simulink model "ssc_car_fuel_cell_1motor"  (R2026a)
settings: Solver=daessc  StopTime=195  FixedStep=1e-3  AbsTol=1e-3
InitFcn:
  | %Vehicle = sm_car_vehcfg_checkConfig(Vehicle);
undefined symbols (not defined in the file): Control, Driver, Init, Maneuver1, Vehicle
libraries: fl_lib x93, nesl_utility x38, GasN_lib x21, sdl_lib x10, simulink_extras x6, SimscapeFluids_lib x6, simulink x5, customMath_lib x5, slpidlib x4, ee_lib x3, autolibshared x2, sl_discontinuities x2
(part 2 of 4)

== system ssc_car_fuel_cell_1motor/Fuel Cell 1 Motor/Regen Torque Limit/Mech to Elec Power Estimate ==
  note: Check if Motoring
      | or Generating
  note: Using an Efficiency Map, we can estimate the
      | Electric Power from the Mechanical  Torque Request.
  note: Pelec_req = Pmech_req*Eff^k,
      | k = -1 if Motoring >= 0,
      | k = 1 if Generating < 0
  MotTrqCmd : Inport
  MotSpd : Inport  Port=2
  Abs : Abs  ZeroCross=off  SaturateOnIntegerOverflow=off
  Abs1 : Abs  ZeroCross=off  SaturateOnIntegerOverflow=off
  Constant1 : Constant  Value=-1  SampleTime=0
  Constant2 : Constant  SampleTime=0
  Eff Map : Lookup_n-D  BreakpointsForDimension1=Control.MotorA1.LossTable.w.Value  BreakpointsForDimension2=Control.MotorA1.LossTable.trq.Value  Table=Control.MotorA1.LossTable.efficiency.Value  ExtrapMethod=Clip  UseLastTableValue=on  InternalRulePriority=Speed  OutDataTypeStr=Inherit: Inherit from 'Table data'  RndMeth=Simplest
      settings: InputPortMap=u0,u1
  Gain1 : Gain  Gain=1/100
  Math Function : Math  Operator=pow  SignedPower=on  OutputSignalType=real
  Product : Product
  Product3 : Product
  Product4 : Product
  Scope : Scope  NumInputPorts=4
      settings: ActiveDisplayYMinimum=84.125  ActiveDisplayYMaximum=92.875  DataLoggingVariableName=ScopeData2
  Switch2 : Switch  ZeroCross=off  SaturateOnIntegerOverflow=off  InputSameDT=off
  rads_to_rpm : Gain  Gain=30/pi
  MotPwrElecReq : Outport  VectorParamsAs1DForOutWhenUnconnected=off
  Eff2k : Outport  Port=2  VectorParamsAs1DForOutWhenUnconnected=off
  wires:
  Product3/1 -> Product4/1
  Switch2/1 -> Math Function/2
  Constant1/1 -> Switch2/1
  Constant2/1 -> Switch2/3
  Eff Map/1 -> Gain1/1, Scope/1
  Abs/1 -> Eff Map/1
  Gain1/1 -> Math Function/1
  Math Function/1 -> Eff2k/1, Product4/2
  Product4/1 -> MotPwrElecReq/1, Scope/2
  Abs1/1 -> Eff Map/2
  rads_to_rpm/1 -> Abs/1
  Product/1 -> Switch2/2
  MotSpd/1 -> Product3/1, Product/1, Scope/3, rads_to_rpm/1
  MotTrqCmd/1 -> Product3/2, Product/2, Scope/4, Abs1/1

== system ssc_car_fuel_cell_1motor/Fuel Cell 1 Motor/Regen Torque Limit/Torque Limit ==
  MotTrq : Inport
  MotSpd : Inport  Port=2
  Gain : Gain  Gain=-1
  MaxMotTrqVsSpd : Lookup_n-D  NumberOfTableDimensions=1  BreakpointsForDimension1=Control.MotorA1.TorqueSpd.w.Value  Table=Control.MotorA1.TorqueSpd.trq.Value  ExtrapMethod=Clip  UseLastTableValue=on  InternalRulePriority=Speed  OutDataTypeStr=Inherit: Inherit from 'Table data'  RndMeth=Simplest
  Saturation Dynamic : sl_discontinuities/Saturation Dynamic  OutMin=[]  OutMax=[]  OutDataTypeStr=Inherit: Same as second input  OutDataType=fixdt(1, 16)  OutScaling=2^-10  DoSatur=off
  rads_to_rpm : Gain  Gain=30/pi
  MotReqCmd : Outport  VectorParamsAs1DForOutWhenUnconnected=off
  wires:
  MotTrq/1 -> Saturation Dynamic/2
  MotSpd/1 -> rads_to_rpm/1
  MaxMotTrqVsSpd/1 -> Gain/1, Saturation Dynamic/1
  rads_to_rpm/1 -> MaxMotTrqVsSpd/1
  Gain/1 -> Saturation Dynamic/3
  Saturation Dynamic/1 -> MotReqCmd/1

== system ssc_car_fuel_cell_1motor/Fuel Cell 1 Motor/Susp/Steer ==
  Bus Creator : BusCreator  Inputs=1
  Constant : Constant  Value=0
  Steer : Outport  VectorParamsAs1DForOutWhenUnconnected=off
  wires:
  Bus Creator/1 -> Steer/1  "Steer"
  Constant/1 -> Bus Creator/1  "iMotor"

== system ssc_car_fuel_cell_1motor/Vehicle/Powertrain/Driveline ==
  Differential : sdl_lib/Gears/Differential  driveshaft_location=2  cd_ratio=Vehicle.Powertrain.Driveline.DifferentialA1.ratio.Value  friction_model=1  efficiency=[.85, .92]  temperature_TLU=[280, 300, 320] K  efficiency_ss_TLU=[.95, .9, .85]  efficiency_cd_TLU=[.95, .9, .85]  pwr_thr=[.001, .001] W  mu_visc=[0, 0] N*m/(rad/s)  model_inertia=0  sun_inertia=1e-10 kg*m^2  sun_radius=0.01 m  carrier_inertia=0.001 kg*m^2  planet_inertia=0.001 kg*m^2  planet_mass=1e-10 kg  thermal_mass=50 J/K  T_init=300 K
  Gear Box : fl_lib/Mechanical/Mechanisms/Gear Box  ratio=Vehicle.Powertrain.Driveline.GearboxA1.ratio.Value  t_in_specify=off  t_in_priority=None  t_in=0 N*m  t_in_nominal_specify=off  t_in_nominal_value=1  t_in_nominal_unit=N*m  t_out_specify=off  t_out_priority=None  t_out=0 N*m  t_out_nominal_specify=off  t_out_nominal_value=1  t_out_nominal_unit=N*m
  Sensor Speed and Power : Subsystem
      mask Display: disp('S')
  Simscape Bus : SimscapeBus  HierarchyStrings=ShaftA1
  L1 : PMIOPort  Side=Left
  Sh : PMIOPort  Port=2  Side=Left
  R1 : PMIOPort  Port=3  Side=Right
  FR1 : PMIOPort  Port=4  Side=Right
  connections:
  Gear Box/LConn1 -- Sensor Speed and Power/RConn1
  Simscape Bus/LConn1 -- Sensor Speed and Power/LConn1
  Differential/RConn2 -- L1/RConn1
  Sh/RConn1 -- Simscape Bus/RConn1
  Differential/RConn1 -- FR1/RConn1 -- R1/RConn1
  Differential/LConn1 -- Gear Box/RConn1

== system ssc_car_fuel_cell_1motor/Vehicle/Powertrain/FuelCell1Motor ==
  In Bus Element : Inport  PortName=CtrlBus  Element=FuelCell
  In Bus Element4 : Inport  PortName=CtrlBus  Element=MotorA1.trqCmd
  In Bus Element1 : Inport  Port=2  PortName=VehBus  Element=Body.CG
  Ambient Temperature : fl_lib/Thermal/Thermal Sources/Temperature Source  temperature=300 K
  Battery : Subsystem  VariantControl=0  mask{Battery=Power.Battery}
      mask prompts: Battery "Battery (structure)"
      mask Display: image('sm_car_vehicle_power_battery_system_IMAGE.png');
  Electrical Reference1 : fl_lib/Electrical/Electrical Elements/Electrical Reference
  Fuel Cell : Subsystem  VariantControl=0  mask{FuelCell=Power.FuelCell}
      mask prompts: FuelCell "Fuel Cell (structure)"
      mask Display: image('sm_car_vehicle_power_fuel_cell_converter_IMAGE.png');
  Motor A1 : Subsystem  mask{Motor=Power.MotorA1}
      mask prompts: Motor "Motor (structure)"
      mask Display: image('sm_car_vehicle_power_emotor_simplified_IMAGE.png');
  Simscape Bus : SimscapeBus  HierarchyStrings=ShaftA1
  Thermal System : Subsystem  mask{Cooling=Power.Cooling}
      mask prompts: Cooling "Cooling (structure)"
      mask Display: image('sm_car_vehicle_power_cooling_active1loop_IMAGE.png');
  Shafts : PMIOPort  Side=Left
  Out Bus Element : Outport  PortName=OutP  Element=FuelCell
  Out Bus Element1 : Outport  PortName=OutP  Element=MotorA1
  Out Bus Element2 : Outport  PortName=OutP  Element=Battery
  Out Bus Element3 : Outport  PortName=OutP  Element=Thermal
  wires:
  Battery/1(m) -> Out Bus Element2/1
  Thermal System/1(m) -> Out Bus Element3/1
  Fuel Cell/1(m) -> Out Bus Element/1
  Motor A1/1(m) -> Out Bus Element1/1
  In Bus Element1/1 -> Fuel Cell/2(VehBus)
  In Bus Element4/1 -> Motor A1/1(Tr)
  In Bus Element/1 -> Fuel Cell/1(CtrlBus)
  Fuel Cell/2(PBatt) -> Battery/1(PLoss)
  connections:
  Motor A1/LConn1 -- Fuel Cell/RConn1 -- Battery/RConn1
  Thermal System/LConn3 -- Battery/RConn4 -- Ambient Temperature/LConn1
  Thermal System/LConn2 -- Fuel Cell/RConn3 -- Battery/RConn3
  Motor A1/LConn3 -- Thermal System/LConn1
  Simscape Bus/RConn1 -- Shafts/RConn1
  Fuel Cell/RConn2 -- Electrical Reference1/LConn1 -- Motor A1/LConn2 -- Battery/RConn2
  Simscape Bus/LConn1 -- Motor A1/RConn1

== system ssc_car_fuel_cell_1motor/Vehicle/Powertrain/Driveline/Sensor Speed and Power ==
  Ideal Rotational Motion Sensor : fl_lib/Mechanical/Mechanical Sensors/Ideal Rotational Motion Sensor  reference=foundation.enum.MeasurementReference.difference  acceleration_port=false  velocity_port=true  position_port=true  wrap_angle=simscape.enum.onoff.off  offset=0 rad
  Ideal Torque Sensor : fl_lib/Mechanical/Mechanical Sensors/Ideal Torque Sensor
  Mechanical Rotational Reference : fl_lib/Mechanical/Rotational Elements/Mechanical Rotational Reference
  PS-Simulink Converter : nesl_utility/PS-Simulink Converter  PhysicalDomain=network_engine_domain  SubClassName=ps_output  LeftPortType=input  RightPortType=output  PseudoPeriodic=off  Frequencies=[]  VectorFormat=1-D array  Unit=N*m  AffineConversion=off
  PS-Simulink Converter1 : nesl_utility/PS-Simulink Converter  PhysicalDomain=network_engine_domain  SubClassName=ps_output  LeftPortType=input  RightPortType=output  PseudoPeriodic=off  Frequencies=[]  VectorFormat=1-D array  Unit=rad/s  AffineConversion=off
  Product : Product  RndMeth=Zero
  Terminator : Terminator
  W2kW : Gain  Gain=0.001
  B : PMIOPort  Side=Left
  F : PMIOPort  Port=2  Side=Right
  wires:
  W2kW/1 -> [Pm_vehicle]
  Product/1 -> W2kW/1
  PS-Simulink Converter/1 -> Product/1
  PS-Simulink Converter1/1 -> Product/2
  [Pm_vehicle] -> Terminator/1
  connections:
  Mechanical Rotational Reference/LConn1 -- Ideal Rotational Motion Sensor/RConn1
  Ideal Rotational Motion Sensor/LConn1 -- F/RConn1 -- Ideal Torque Sensor/RConn1
  B/RConn1 -- Ideal Torque Sensor/LConn1
  PS-Simulink Converter/LConn1 -- Ideal Torque Sensor/RConn2
  PS-Simulink Converter1/LConn1 -- Ideal Rotational Motion Sensor/RConn2

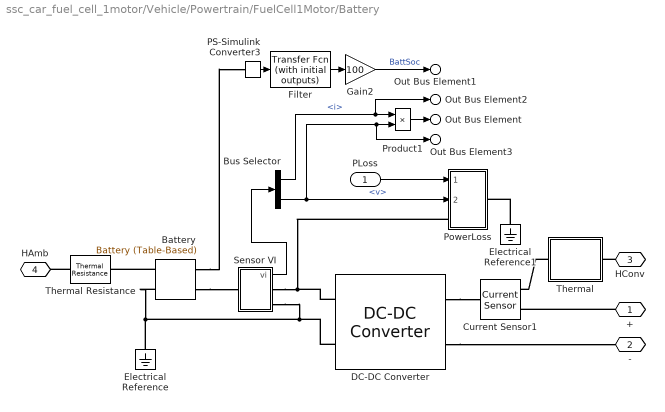
== system ssc_car_fuel_cell_1motor/Vehicle/Powertrain/FuelCell1Motor/Battery ==
  PLoss : Inport
  Battery : batteryecm_lib/Battery (Table-Based)  SOC_vec=Battery.vNoLoad.SOC.Value  T_dependence=simscape.enum.tablebattery.temperature_dependence.yes  prm_dir=simscape.enum.tablebattery.prm_dir.noCurrentDirectionality  T_vec=Battery.vNoLoad.T.Value K  V0_mat=Battery.vNoLoad.V0.Value V  V0_vec=[3.1, 3.27, 3.31, 3.5] V  V_range=[0, inf] V  R0_mat=Battery.rTerminal.R0.Value Ohm  R0_vec=[.015, .017, .012, .013] Ohm  R0_dis_mat=[.03, .015, .002; .04, .017, .008; .039, .012, .006; .027, .013, .021] Ohm  R0_dis_vec=[.015, .017, .012, .013] Ohm  R0_ch_mat=[.03, .015, .002; .04, .017, .008; .039, .012, .006; .027, .013, .021] Ohm  R0_ch_vec=[.015, .017, .012, .013] Ohm  AH=Battery.AhTable.Ah.Value hr*A  prm_leak=1  Rleak_vec=ones(size(Battery.vNoLoad.T.Value))*10000 Ohm  Rleak=7e3 Ohm  extrapolation_option=simscape.enum.extrapolation.linear  SOC_port=simscape.enum.tablebattery.enable.yes  prm_dyn=1  R1_mat=[.089, .076, .01; .042, .022, .099; .019, .007, .002; .051, .043, .029] Ohm  R1_vec=[.076, .022, .007, .043] Ohm  tau1_mat=[44, 148, 235; 93, 110, 1000; 19, 27, 133; .5, 22, 3] s  tau1_vec=[148, 110, 27, 22] s  R2_mat=[.014, .382, .407; .028, .006, .007; .014, .007, .006; .333, .956, .912] Ohm  R2_vec=[.382, .006, .007, .956] Ohm  tau2_mat=[1, 44, 5644; 11, 24, 506; 2, 14, 330; 3310, 13419, 30216] s  tau2_vec=[44, 24, 14, 13419] s  R3_mat=[.014, .382, .407; .028, .006, .007; .014, .007, .006; .333, .956, .912] Ohm  R3_vec=[.382, .006, .007, .956] Ohm  tau3_mat=[1, 44, 5644; 11, 24, 506; 2, 14, 330; 3310, 13419, 30216] s  tau3_vec=[44, 24, 14, 13419] s  R4_mat=[.014, .382, .407; .028, .006, .007; .014, .007, .006; .333, .956, .912] Ohm  R4_vec=[.382, .006, .007, .956] Ohm  tau4_mat=[1, 44, 5644; 11, 24, 506; 2, 14, 330; 3310, 13419, 30216] s  tau4_vec=[44, 24, 14, 13419] s  R5_mat=[.014, .382, .407; .028, .006, .007; .014, .007, .006; .333, .956, .912] Ohm  R5_vec=[.382, .006, .007, .956] Ohm  tau5_mat=[1, 44, 5644; 11, 24, 506; 2, 14, 330; 3310, 13419, 30216] s  tau5_vec=[44, 24, 14, 13419] s  prm_fade=simscape.enum.tablebattery.prm_fade.equations  N0=100  dV0=0  dR0=0  dAH=0  dRleak=0  dR1=0  dR2=0  dR3=0  dR4=0  dR5=0  N0vec=[100, 200, 300]  Tfadevec=[298.15, 323.15] K  dV0vec=[0, 0, 0]  dR0vec=[0, 0, 0]  dAHvec=[0, 0, 0]  dRleakvec=[0, 0, 0]  dR1vec=[0, 0, 0]  dR2vec=[0, 0, 0]  dR3vec=[0, 0, 0]  dR4vec=[0, 0, 0]  dR5vec=[0, 0, 0]  dV0mat=[0, 0; 0, 0; 0, 0]  dR0mat=[0, 0; 0, 0; 0, 0]  dAHmat=[0, 0; 0, 0; 0, 0]  dRleakmat=[0, 0; 0, 0; 0, 0]  dR1mat=[0, 0; 0, 0; 0, 0]  dR2mat=[0, 0; 0, 0; 0, 0]  dR3mat=[0, 0; 0, 0; 0, 0]  dR4mat=[0, 0; 0, 0; 0, 0]  dR5mat=[0, 0; 0, 0; 0, 0]  prm_age_modeling=simscape.enum.tablebattery.prm_age_modeling.equation  storage_dt_age_vec=[0] d  storage_T_age_vec=[273] K  prm_age_OCV=simscape.enum.tablebattery.prm_age_OCV.OCV  OCV_age=0.9  SOC_age=0.6  prm_age_resistance=simscape.enum.tablebattery.prm_age.disabled  OCV_scaling_age_resistance=2.2134e6  OCV_offset_age_resistance=1.632e6  temp_exp_age_resistance=0.515833569 V  t_exp_age_resistance=0.75  T_age_vec_resistance=[273.15, 298.15, 323.15] K  dt_age_vec_resistance=[90, 180, 270, 360] d  dR0_age_vec=[0, 0, 0]  t_meas_dR0_age=100 d  dR0_age_mat=[0, 0, 0; 0, 0, 0; 0, 0, 0; 0, 0, 0]  prm_age_capacity=simscape.enum.tablebattery.prm_age.disabled  OCV_scaling_age_capacity=1.5097e07  OCV_offset_age_capacity=8.3625e06  temp_exp_age_capacity=0.6011 V  t_exp_age_capacity=0.75  T_age_vec_capacity=[273.15, 298.15, 323.15] K  dt_age_vec_capacity=[90, 180, 270, 360] d  dAH_age_vec=[0, 0, 0]  t_meas_dAH_age=100 d  dAH_age_mat=[0, 0, 0; 0, 0, 0; 0, 0, 0; 0, 0, 0]  thermal_port=simscape.enum.thermaleffects.model  temperature=Battery.TInit.Value K  thermal_mass=Battery.mThermal.Value J/K  i_specify=on  i_priority=None  i=1e-3 A  i_nominal_specify=off  i_nominal_value=1  i_nominal_unit=A  v_specify=off  v_priority=None  v=0 V  v_nominal_specify=off  v_nominal_value=1  v_nominal_unit=V  stateOfCharge_specify=on  stateOfCharge_priority=High  stateOfCharge=Battery.SOCInit.Value  stateOfCharge_nominal_specify=off  stateOfCharge_nominal_value=1  stateOfCharge_nominal_unit=1  num_cycles_specify=off  num_cycles_priority=High  num_cycles=0  num_cycles_nominal_specify=off  num_cycles_nominal_value=1  num_cycles_nominal_unit=1  cell_temperature_specify=on  cell_temperature_priority=High  cell_temperature=Battery.TInit.Value K  cell_temperature_nominal_specify=off  cell_temperature_nominal_value=1  cell_temperature_nominal_unit=K
  Bus Selector : BusSelector  OutputSignals=i,v
  Current Sensor1 : fl_lib/Electrical/Electrical Sensors/Current Sensor
  DC-DC Converter : ee_lib/Semiconductors & Converters/Converters/DC-DC Converter  Vref_option=ee.enum.converters.voltageref.internal  v_ref="Battery.Converter.vRef.Value  V"  P_rated=Battery.Converter.power.Value W  droop_enabled=true  droop_param=1  droop=Battery.Converter.droopVpA.Value V/A  droop_percent=2  Vref_droop=10 V  reversible=1  G_diode=1e-6 1/Ohm  P_fixed=Battery.Converter.lossFixed.Value W  losses_option=ee.enum.converters.lossesOption.proportionalToSquaredCurrent  eff_rated=80  tableOption=ee.enum.converters.lossTableOption.current  i_eff_vec=[1, 2, 3, 4] A  v_eff_vec=[15, 30, 45] V  eff_vec=[90, 80, 70, 60]  eff_2D_table=[90, 85, 80; 80, 75, 70; 70, 65, 60; 60, 55, 50]  model_dynamics=0  tau=0.02 s  v_ini=650 V  v1_min=1 V  R1=1000 Ohm  R2=1000 Ohm  T_eff_vec=[280, 300, 320] K  eff_3D_table=repmat([66; 76; 80; 74], 1, 3, 3)  thermal_mass=100 J/K  initial_temperature=298.15 K
  Electrical Reference : fl_lib/Electrical/Electrical Elements/Electrical Reference
  Electrical Reference1 : fl_lib/Electrical/Electrical Elements/Electrical Reference
  Filter : simulink_extras/Additional Linear/Transfer Fcn (with initial outputs)  N=[1]  D=[.01 1]  Y0=Battery.SOCInit.Value  U0=0
  Gain2 : Gain  Gain=100
  PS-Simulink Converter3 : nesl_utility/PS-Simulink Converter  PhysicalDomain=network_engine_domain  SubClassName=ps_output  LeftPortType=input  RightPortType=output  PseudoPeriodic=off  Frequencies=[]  VectorFormat=1-D array  Unit=1  AffineConversion=off
  PowerLoss : Subsystem
  Product1 : Product
  Sensor VI : Subsystem
  Thermal : Subsystem
  Thermal Resistance : fl_lib/Thermal/Thermal Elements/Thermal Resistance  resistance=Battery.rThermal.Value K/W  T_specify=off  T_priority=None  T=0 K  T_nominal_specify=off  T_nominal_value=1  T_nominal_unit=K  Q_specify=off  Q_priority=None  Q=0 W  Q_nominal_specify=off  Q_nominal_value=1  Q_nominal_unit=W
  + : PMIOPort  Side=Right
  - : PMIOPort  Port=2  Side=Right
  HConv : PMIOPort  Port=3  Side=Right
  HAmb : PMIOPort  Port=4  Side=Right
  Out Bus Element : Outport  PortName=m  Element=Power
  Out Bus Element1 : Outport  PortName=m  Element=SOC
  Out Bus Element2 : Outport  PortName=m  Element=i
  Out Bus Element3 : Outport  PortName=m  Element=v
  wires:
  Sensor VI/1(vi) -> Bus Selector/1
  Product1/1 -> Out Bus Element/1
  Bus Selector/1 -> Out Bus Element2/1, Product1/1  "<i>"
  PLoss/1 -> PowerLoss/1(PLoss)
  Bus Selector/2 -> PowerLoss/2(VBatt), Out Bus Element3/1, Product1/2  "<v>"
  Filter/1 -> Gain2/1
  Gain2/1 -> Out Bus Element1/1  "BattSoc"
  PS-Simulink Converter3/1 -> Filter/1
  connections:
  Thermal/LConn1 -- Current Sensor1/RConn1
  HConv/RConn1 -- Thermal/RConn1
  Electrical Reference1/LConn1 -- PowerLoss/RConn1
  Thermal Resistance/LConn1 -- HAmb/RConn1
  DC-DC Converter/RConn1 -- Current Sensor1/LConn1
  DC-DC Converter/RConn2 -- -/RConn1
  +/RConn1 -- Current Sensor1/RConn2
  Battery/RConn2 -- Thermal Resistance/RConn1
  Sensor VI/RConn2 -- DC-DC Converter/LConn2 -- Battery/RConn1 -- Electrical Reference/LConn1
  Battery/LConn1 -- Sensor VI/LConn1
  Battery/LConn2 -- PS-Simulink Converter3/LConn1
  Sensor VI/RConn1 -- DC-DC Converter/LConn1 -- PowerLoss/LConn1

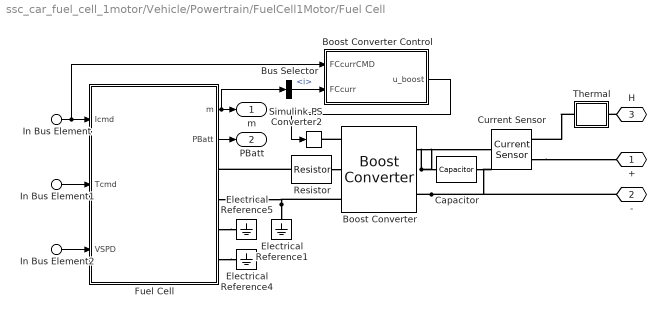
== system ssc_car_fuel_cell_1motor/Vehicle/Powertrain/FuelCell1Motor/Fuel Cell ==
  In Bus Element : Inport  PortName=CtrlBus  Element=iCmd
  In Bus Element1 : Inport  PortName=CtrlBus  Element=TFuelCellCmd
  In Bus Element2 : Inport  Port=2  PortName=VehBus  Element=vx
  Boost Converter : ee_lib/Semiconductors & Converters/Converters/Boost Converter  port_option=ee.enum.controlport.ps  device_type=ee.enum.converters.switchingdevice.averaged  Vf=0.8 V  Ron=FuelCell.ConverterB.rOn.Value Ohm  Rds=0.001 Ohm  Goff=1e-5 1/Ohm  Vgt=1 V  Vgt_off=-1 V  Ih=1 A  Vth=6 V  K=0  diode_param=ee.enum.converters.diode.nodynamics  diode_Vf=FuelCell.ConverterB.Diode.vForward.Value V  diode_Ron=FuelCell.ConverterB.Diode.rOn.Value Ohm  diode_Goff=FuelCell.ConverterB.Diode.GOff.Value 1/Ohm  diode_C=50 nF  diode_iRM=-235 A  diode_iF=300 A  diode_idot=-50 A/us  diode_trr_param=ee.enum.converters.diodetrr.trr_factor  diode_trr_factor=3  diode_trr=15 us  diode_Qrr=1500 s*uA  Lf=FuelCell.ConverterB.Lint.L.Value H  Rl=0 Ohm  Cf=FuelCell.ConverterB.Cint.C.Value F  Rf=FuelCell.ConverterB.Cint.r.Value Ohm  snubber_type=ee.enum.converters.snubber.exclude  Cs=1e-7 F  Rs=0.1 Ohm  iL_specify=on  iL_priority=Low  iL=0 A  iL_nominal_specify=off  iL_nominal_value=1  iL_nominal_unit=A  vc_specify=on  vc_priority=Low  vc=FuelCell.Converter.vRef.Value V  vc_nominal_specify=off  vc_nominal_value=1  vc_nominal_unit=V
  Boost Converter Control : Subsystem
  Bus Selector : BusSelector  OutputSignals=i
  Capacitor : fl_lib/Electrical/Electrical Elements/Capacitor  c=FuelCell.ConverterB.Cext.C.Value F  r=FuelCell.ConverterB.Cext.r.Value Ohm  g=FuelCell.ConverterB.Cext.G.Value 1/Ohm  i_specify=off  i_priority=None  i=0 A  i_nominal_specify=off  i_nominal_value=1  i_nominal_unit=A  v_specify=off  v_priority=None  v=0 V  v_nominal_specify=off  v_nominal_value=1  v_nominal_unit=V  vc_specify=on  vc_priority=Low  vc=FuelCell.Converter.vRef.Value V  vc_nominal_specify=off  vc_nominal_value=1  vc_nominal_unit=V
  Current Sensor : fl_lib/Electrical/Electrical Sensors/Current Sensor
  Electrical Reference1 : fl_lib/Electrical/Electrical Elements/Electrical Reference
  Electrical Reference4 : fl_lib/Electrical/Electrical Elements/Electrical Reference
  Electrical Reference5 : fl_lib/Electrical/Electrical Elements/Electrical Reference
  Fuel Cell : Subsystem
      mask Display: image('sm_car_vehicle_power_fuel_cell_IMAGE.png');
  Resistor : fl_lib/Electrical/Electrical Elements/Resistor  R=FuelCell.ConverterB.Lint.r.Value Ohm  i_specify=off  i_priority=None  i=0 A  i_nominal_specify=off  i_nominal_value=1  i_nominal_unit=A  v_specify=off  v_priority=None  v=0 V  v_nominal_specify=off  v_nominal_value=1  v_nominal_unit=V
  Simulink-PS Converter2 : nesl_utility/Simulink-PS Converter  PhysicalDomain=network_engine_domain  SubClassName=ps_input  LeftPortType=input  RightPortType=output  PseudoPeriodic=off  Frequencies=[]  NoiseDistribution=none  NoiseParameters=[]  Unit=1  AffineConversion=off  FilteringAndDerivatives=provide  SimscapeFilterOrder=1  InputFilterTimeConstant=0.001  UdotUserProvided=0
  Thermal : Subsystem
  + : PMIOPort  Side=Right
  - : PMIOPort  Port=2  Side=Right
  H : PMIOPort  Port=3  Side=Right
  m : Outport
  PBatt : Outport  Port=2
  wires:
  Bus Selector/1 -> Boost Converter Control/2(FCcurr)  "<i>"
  Boost Converter Control/1(u_boost) -> Simulink-PS Converter2/1
  In Bus Element/1 -> Fuel Cell/1(Icmd), Boost Converter Control/1(FCcurrCMD)
  Fuel Cell/2(PBatt) -> PBatt/1
  Fuel Cell/1(m) -> m/1, Bus Selector/1
  In Bus Element1/1 -> Fuel Cell/2(Tcmd)
  In Bus Element2/1 -> Fuel Cell/3(VSPD)
  connections:
  Resistor/RConn1 -- Boost Converter/LConn2
  Boost Converter/RConn2 -- Capacitor/RConn1 -- -/RConn1
  Boost Converter/LConn1 -- Simulink-PS Converter2/RConn1
  Capacitor/LConn1 -- Current Sensor/LConn1 -- Boost Converter/RConn1
  Thermal/LConn1 -- Current Sensor/RConn1
  H/RConn1 -- Thermal/RConn1
  Resistor/LConn1 -- Fuel Cell/RConn1
  Fuel Cell/RConn4 -- Electrical Reference4/LConn1
  Fuel Cell/RConn3 -- Electrical Reference5/LConn1
  Current Sensor/RConn2 -- +/RConn1
  Electrical Reference1/LConn1 -- Boost Converter/LConn3 -- Fuel Cell/RConn2

== system ssc_car_fuel_cell_1motor/Vehicle/Powertrain/FuelCell1Motor/Motor A1 ==
  note: This resistor is here to guide model initialization.
  Tr : Inport
  Mechanical Rotational Reference : fl_lib/Mechanical/Rotational Elements/Mechanical Rotational Reference
  Motor : ee_lib/Electromechanical/Motor & Drive (System Level)  torque_speed_param=1  overtorque_param=ee.enum.electromech.overtorque.no  T_t=Motor.TorqueSpd.trq.Value N*m  T_t_intermittent=[.36, .32, .28, 0] N*m  T_t_2D=[.09, .09, .09; .08, .08, .08; .07, .07, .07; 0, 0, 0] N*m  T_t_intermittent_2D=[.36, .36, .36; .32, .32, .32; .28, .28, .28; 0, 0, 0] N*m  w_t=Motor.TorqueSpd.w.Value rpm  vdc_t=[6, 12, 24] V  torque_max=0.1 N*m  power_max=30 W  torque_max_intermittent=0.4 N*m  power_max_intermittent=120 W  time_overtorque=30 s  time_recover=60 s  Tc=1/Motor.fActuatorCutoff.Value s  EnableSwitch=simscape.enum.onoff.off  losses_param=3  eff=100  w_eff=3750 rpm  T_eff=0.08 N*m  Piron=0 W  Pbase=0 W  w_eff_vec=Motor.TorqueSpd.w.Value rpm  T_eff_vec=Motor.LossTable.trq.Value N*m  v_eff_vec=[100, 250, 400] V  losses_mat=[1.49, 1.67, 2.21, 3.1; .42, .69, 1.14, 2.03; .06, .24, .78, 1.68; .42, .69, 1.14, 2.03; 1.49, 1.67, 2.21, 3.1] W  efficiency_mat=Motor.LossTable.efficiency.Value  losses_mat_3D=ones(5, 4, 3) W  efficiency_mat_3D=95 * ones(5, 4, 3)  Res=Motor.Rsupply.Value Ohm  J=Motor.J.Value kg*m^2  lam=Motor.b.Value N*m/(rad/s)  speed0=0 rpm  faulted_specify=off  faulted_priority=None  faulted=0  faulted_nominal_specify=off  faulted_nominal_value=1  faulted_nominal_unit=1  isSwitchedOff_specify=off  isSwitchedOff_priority=None  isSwitchedOff=0  isSwitchedOff_nominal_specify=off  isSwitchedOff_nominal_value=1  isSwitchedOff_nominal_unit=1  torqueLimitContinuous_specify=off  torqueLimitContinuous_priority=None  torqueLimitContinuous=0 N*m  torqueLimitContinuous_nominal_specify=off  torqueLimitContinuous_nominal_value=1  torqueLimitContinuous_nominal_unit=N*m  TabulateLossesForMultipleTemperatures=false  alpha=3.93e-3 1/K  Tmeas=Motor.ThermalLoss.T1.Value degC  TmeasVec=[25, 75, 125] degC  Tmeas2=Motor.ThermalLoss.T2.Value degC  losses_mat_T2=[1.49, 1.74, 2.49, 3.74; .42, .67, 1.42, 2.67; .06, .31, 1.06, 2.31; .42, .67, 1.42, 2.67; 1.49, 1.74, 2.49, 3.74] W  efficiency_mat_T2=Motor.ThermalLoss.efficiency.Value  losses_mat_3D_T2=ones(5, 4, 3) W  efficiency_mat_3D_T2=95 * ones(5, 4, 3)  lossesMatMultipleTemperatures=ones(5, 4, 3) W  efficiencyMatMultipleTemperatures=95 * ones(5, 4, 3)  lossesMat4DMultipleTemperatures=ones(5, 4, 3, 3) W  efficiencyMat4DMultipleTemperatures=95 * ones(5, 4, 3, 3)  thermal_mass=Motor.ThermalLoss.mThermal.Value J/K  initial_temperature=Motor.ThermalLoss.Tinit.Value K
  PS-Simulink Converter2 : nesl_utility/PS-Simulink Converter  PhysicalDomain=network_engine_domain  SubClassName=ps_output  LeftPortType=input  RightPortType=output  PseudoPeriodic=off  Frequencies=[]  VectorFormat=1-D array  Unit=rad/s  AffineConversion=off
  Resistor : fl_lib/Electrical/Electrical Elements/Resistor  R=1e-6 Ohm  i_specify=on  i_priority=High  i=0.1*Init.Axle1.nWheel.Value(1) A  i_nominal_specify=off  i_nominal_value=1  i_nominal_unit=A  v_specify=off  v_priority=None  v=0 V  v_nominal_specify=off  v_nominal_value=1  v_nominal_unit=V
  Sensing Current : Subsystem
  Sensing Torque : Subsystem
  Simulink-PS Converter2 : nesl_utility/Simulink-PS Converter  PhysicalDomain=network_engine_domain  SubClassName=ps_input  LeftPortType=input  RightPortType=output  PseudoPeriodic=off  Frequencies=[]  NoiseDistribution=none  NoiseParameters=[]  Unit=N*m  AffineConversion=off  FilteringAndDerivatives=provide  SimscapeFilterOrder=1  InputFilterTimeConstant=0.001  UdotUserProvided=0
  + : PMIOPort  Side=Left
  - : PMIOPort  Port=2  Side=Left
  R : PMIOPort  Port=3  Side=Right
  H : PMIOPort  Port=4  Side=Left
  Out Bus Element : Outport  PortName=m  Element=w
  Out Bus Element1 : Outport  PortName=m  Element=i
  Out Bus Element2 : Outport  PortName=m  Element=trq
  wires:
  Sensing Torque/1(trq) -> Out Bus Element2/1
  Sensing Current/1(i) -> Out Bus Element1/1
  Tr/1 -> Simulink-PS Converter2/1
  PS-Simulink Converter2/1 -> Out Bus Element/1
  connections:
  +/RConn1 -- Resistor/RConn1
  Sensing Torque/RConn1 -- R/RConn1
  Sensing Current/RConn1 -- Resistor/LConn1
  Motor/RConn2 -- PS-Simulink Converter2/LConn1
  Motor/RConn3 -- H/RConn1
  Motor/RConn1 -- -/RConn1
  Motor/LConn1 -- Sensing Current/LConn1
  Motor/LConn3 -- Sensing Torque/LConn1
  Motor/LConn2 -- Simulink-PS Converter2/RConn1
  Motor/RConn4 -- Mechanical Rotational Reference/LConn1

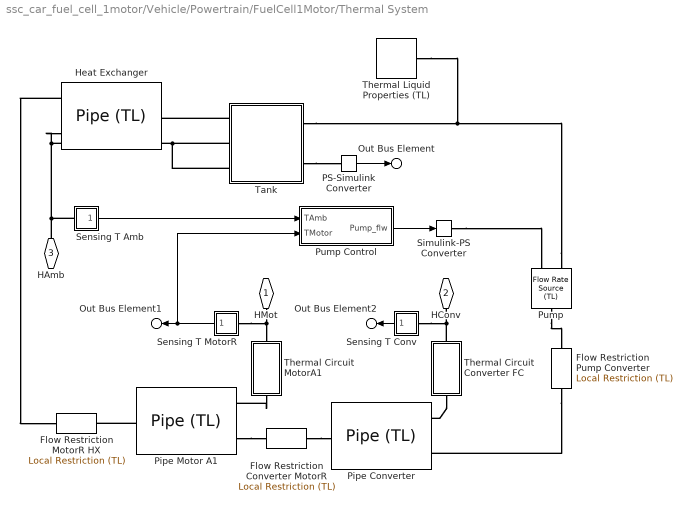
== system ssc_car_fuel_cell_1motor/Vehicle/Powertrain/FuelCell1Motor/Thermal System ==
  Flow Restriction Converter MotorR : fl_lib/Thermal Liquid/Elements/Local Restriction (TL)  restriction_type=foundation.enum.restriction_type.fixed  restriction_area=Cooling.Restriction.area.Value m^2  min_area=1e-10 m^2  max_area=0.005 m^2  area=Cooling.Restriction.areaPorts.Value m^2  Cd=Cooling.Restriction.dischargeCoeff.Value  Re_c=Cooling.Restriction.CriticalReynolds.Value  pressure_recovery=simscape.enum.onoff.on
  Flow Restriction MotorR HX : fl_lib/Thermal Liquid/Elements/Local Restriction (TL)  restriction_type=foundation.enum.restriction_type.fixed  restriction_area=Cooling.Restriction.area.Value m^2  min_area=1e-10 m^2  max_area=0.005 m^2  area=Cooling.Restriction.areaPorts.Value m^2  Cd=Cooling.Restriction.dischargeCoeff.Value  Re_c=Cooling.Restriction.CriticalReynolds.Value  pressure_recovery=simscape.enum.onoff.on
  Flow Restriction Pump Converter : fl_lib/Thermal Liquid/Elements/Local Restriction (TL)  restriction_type=foundation.enum.restriction_type.fixed  restriction_area=Cooling.Restriction.area.Value m^2  min_area=1e-10 m^2  max_area=0.005 m^2  area=Cooling.Restriction.areaPorts.Value m^2  Cd=Cooling.Restriction.dischargeCoeff.Value  Re_c=Cooling.Restriction.CriticalReynolds.Value  pressure_recovery=simscape.enum.onoff.on
  Heat Exchanger : SimscapeFluids_lib/Thermal Liquid/Pipes & Fittings/Pipe (TL)  dynamic_compressibility=0  inertia=0  num_segments=1  pipe_length=Cooling.HX.x.Value m  cross_section_geometry=fluids.thermal_liquid.pipes_fittings.enum.CrossSectionGeometry.Custom  pipe_diameter=0.1 m  pipe_inner_diameter=0.05 m  pipe_outer_diameter=0.1 m  pipe_width=0.1 m  pipe_height=0.1 m  pipe_major_axis=0.1 m  pipe_minor_axis=0.05 m  pipe_side=0.1 m  pipe_angle=30 deg  area=Cooling.HX.area.Value m^2  Dh=Cooling.HX.diameter.Value m  elevation_spec=foundation.enum.constant_variable.constant  elevation_gain=Cooling.HX.elevation.Value m  gravity_spec=foundation.enum.constant_variable.constant  g=9.81 m/s^2  pressure_loss_spec=1  local_pressure_loss_spec=fluids.thermal_liquid.pipes_fittings.enum.LocalLossSpec.AggregateLength  length_add=Cooling.HX.xResistance.Value m  loss_coefficient=0.1  roughness_spec=fluids.thermal_liquid.pipes_fittings.enum.RoughnessSpec.Custom  roughness=Cooling.HX.roughness.Value m  Re_friction_TLU=[ 400 1000 1.5e+3 3e+3 4e+3 6e+3 1e+4 2e+4 4e+4 6e+4 1e+5 1e+8 ]  friction_factor_TLU=[ 0.264 0.112 0.07099999999999999 0.0417 0.0387 0.0268 0.025 0.0232 0.0226 0.022 0.0214 0.0214 ]  Re_lam=Cooling.HX.laminarReynoldsMax.Value  Re_tur=Cooling.HX.turbulentReynoldsMin.Value  shape_factor=Cooling.HX.frictionDarcy.Value  mdot_nominal=[ 0.1 1 ] kg/s  p_diff_nominal=[ 0.001 0.01 ] MPa  mdot_threshold=1e-6 kg/s  wall_spec=1  vol_expansion_spec=fluids.thermal_liquid.pipes_fittings.enum.VolumeExpansionSpec.Diameter  area_pressure_gain=1e-6 m^2/MPa  static_pressure_TLU=[.1, 1] MPa  area_pressure_gain_TLU=[1e-05, 1.1e-05] m^2  material_behavior_spec=fluids.thermal_liquid.pipes_fittings.enum.PipeMaterialBehavior.Linear  diameter_pressure_gain=1.2e-6 m/MPa  wall_thickness=0.05 m  elastic_modulus=69 GPa  stress_TLU=[276, 310] MPa  strain_TLU=[.004, .02]  stress_assert_action=simscape.enum.assert.action.none  stress_max=400 MPa  poisson_ratio=0.33  wall_time_constant=0.01 s  thermal_expansion=false  alpha_L_wall=24 um/(deltaK*m)  thermal_expansion_Tref=293.15 K  heat_transfer_spec=1  mdot_nominal_heat=[ 0.1 1 ] kg/s  T_in_nominal=[ 293.15 293.15 ] K  T_out_nominal=[ 300 300 ] K  p_in_nominal_heat=[ 0.101325 0.101325 ] MPa  T_wall_nominal=[ 303.15 303.15 ] K  a_coeff=0.023  b_Re_power=0.8  c_Pr_power=0.4  Nu_lam=Cooling.HX.laminarNusselt.Value  Re_Colburn_TLU=[ 100 150 1000 ]  Colburn_factor_TLU=[ 0.019 0.013 0.002 ]  Re_Nu_TLU=[ 100 150 1000 ]  Pr_Nu_TLU=[ 1 10 ]  Nu_TLU=[ 3.72 4.21; 3.75 4.44; 4.21 7.15 ]  p0_vec=0.101325 MPa  T0_vec=300 K  mdot0=0.1 kg/s  p_nominal=0.101325 MPa  T_nominal=293.15 K
  PS-Simulink Converter : nesl_utility/PS-Simulink Converter  PhysicalDomain=network_engine_domain  SubClassName=ps_output  LeftPortType=input  RightPortType=output  PseudoPeriodic=off  Frequencies=[]  VectorFormat=1-D array  Unit=K  AffineConversion=off
  Pipe Converter : SimscapeFluids_lib/Thermal Liquid/Pipes & Fittings/Pipe (TL)  dynamic_compressibility=0  inertia=0  num_segments=1  pipe_length=Cooling.Converter.Pipe.x.Value m  cross_section_geometry=fluids.thermal_liquid.pipes_fittings.enum.CrossSectionGeometry.Custom  pipe_diameter=0.1 m  pipe_inner_diameter=0.05 m  pipe_outer_diameter=0.1 m  pipe_width=0.1 m  pipe_height=0.1 m  pipe_major_axis=0.1 m  pipe_minor_axis=0.05 m  pipe_side=0.1 m  pipe_angle=30 deg  area="Cooling.Converter.Pipe.area.Value  m^2"  Dh=Cooling.Converter.Pipe.diameter.Value m  elevation_spec=foundation.enum.constant_variable.constant  elevation_gain=Cooling.Converter.Pipe.elevation.Value m  gravity_spec=foundation.enum.constant_variable.constant  g=9.81 m/s^2  pressure_loss_spec=1  local_pressure_loss_spec=fluids.thermal_liquid.pipes_fittings.enum.LocalLossSpec.AggregateLength  length_add=Cooling.Converter.Pipe.xResistance.Value m  loss_coefficient=0.1  roughness_spec=fluids.thermal_liquid.pipes_fittings.enum.RoughnessSpec.Custom  roughness=Cooling.Converter.Pipe.roughness.Value m  Re_friction_TLU=[ 400 1000 1.5e+3 3e+3 4e+3 6e+3 1e+4 2e+4 4e+4 6e+4 1e+5 1e+8 ]  friction_factor_TLU=[ 0.264 0.112 0.07099999999999999 0.0417 0.0387 0.0268 0.025 0.0232 0.0226 0.022 0.0214 0.0214 ]  Re_lam=Cooling.Converter.Pipe.laminarReynoldsMax.Value  Re_tur=Cooling.Converter.Pipe.turbulentReynoldsMin.Value  shape_factor=Cooling.Converter.Pipe.frictionDarcy.Value  mdot_nominal=[ 0.1 1 ] kg/s  p_diff_nominal=[ 0.001 0.01 ] MPa  mdot_threshold=1e-6 kg/s  wall_spec=1  vol_expansion_spec=fluids.thermal_liquid.pipes_fittings.enum.VolumeExpansionSpec.Diameter  area_pressure_gain=1e-6 m^2/MPa  static_pressure_TLU=[.1, 1] MPa  area_pressure_gain_TLU=[1e-05, 1.1e-05] m^2  material_behavior_spec=fluids.thermal_liquid.pipes_fittings.enum.PipeMaterialBehavior.Linear  diameter_pressure_gain=1.2e-6 m/MPa  wall_thickness=0.05 m  elastic_modulus=69 GPa  stress_TLU=[276, 310] MPa  strain_TLU=[.004, .02]  stress_assert_action=simscape.enum.assert.action.none  stress_max=400 MPa  poisson_ratio=0.33  wall_time_constant=0.01 s  thermal_expansion=false  alpha_L_wall=24 um/(deltaK*m)  thermal_expansion_Tref=293.15 K  heat_transfer_spec=1  mdot_nominal_heat=[ 0.1 1 ] kg/s  T_in_nominal=[ 293.15 293.15 ] K  T_out_nominal=[ 300 300 ] K  p_in_nominal_heat=[ 0.101325 0.101325 ] MPa  T_wall_nominal=[ 303.15 303.15 ] K  a_coeff=0.023  b_Re_power=0.8  c_Pr_power=0.4  Nu_lam=Cooling.Converter.Pipe.laminarNusselt.Value  Re_Colburn_TLU=[ 100 150 1000 ]  Colburn_factor_TLU=[ 0.019 0.013 0.002 ]  Re_Nu_TLU=[ 100 150 1000 ]  Pr_Nu_TLU=[ 1 10 ]  Nu_TLU=[ 3.72 4.21; 3.75 4.44; 4.21 7.15 ]  p0_vec=0.101325 MPa  T0_vec=300 K  mdot0=0.1 kg/s  p_nominal=0.101325 MPa  T_nominal=293.15 K
  Pipe Motor A1 : SimscapeFluids_lib/Thermal Liquid/Pipes & Fittings/Pipe (TL)  dynamic_compressibility=0  inertia=0  num_segments=1  pipe_length=Cooling.MotorA1.Pipe.x.Value m  cross_section_geometry=fluids.thermal_liquid.pipes_fittings.enum.CrossSectionGeometry.Custom  pipe_diameter=0.1 m  pipe_inner_diameter=0.05 m  pipe_outer_diameter=0.1 m  pipe_width=0.1 m  pipe_height=0.1 m  pipe_major_axis=0.1 m  pipe_minor_axis=0.05 m  pipe_side=0.1 m  pipe_angle=30 deg  area=Cooling.MotorA1.Pipe.area.Value m^2  Dh=Cooling.MotorA1.Pipe.diameter.Value m  elevation_spec=foundation.enum.constant_variable.constant  elevation_gain=Cooling.MotorA1.Pipe.elevation.Value m  gravity_spec=foundation.enum.constant_variable.constant  g=9.81 m/s^2  pressure_loss_spec=1  local_pressure_loss_spec=fluids.thermal_liquid.pipes_fittings.enum.LocalLossSpec.AggregateLength  length_add=Cooling.MotorA1.Pipe.xResistance.Value m  loss_coefficient=0.1  roughness_spec=fluids.thermal_liquid.pipes_fittings.enum.RoughnessSpec.Custom  roughness=Cooling.MotorA1.Pipe.roughness.Value m  Re_friction_TLU=[ 400 1000 1.5e+3 3e+3 4e+3 6e+3 1e+4 2e+4 4e+4 6e+4 1e+5 1e+8 ]  friction_factor_TLU=[ 0.264 0.112 0.07099999999999999 0.0417 0.0387 0.0268 0.025 0.0232 0.0226 0.022 0.0214 0.0214 ]  Re_lam=Cooling.MotorA1.Pipe.laminarReynoldsMax.Value  Re_tur=Cooling.MotorA1.Pipe.turbulentReynoldsMin.Value  shape_factor=Cooling.MotorA1.Pipe.frictionDarcy.Value  mdot_nominal=[ 0.1 1 ] kg/s  p_diff_nominal=[ 0.001 0.01 ] MPa  mdot_threshold=1e-6 kg/s  wall_spec=1  vol_expansion_spec=fluids.thermal_liquid.pipes_fittings.enum.VolumeExpansionSpec.Diameter  area_pressure_gain=1e-6 m^2/MPa  static_pressure_TLU=[.1, 1] MPa  area_pressure_gain_TLU=[1e-05, 1.1e-05] m^2  material_behavior_spec=fluids.thermal_liquid.pipes_fittings.enum.PipeMaterialBehavior.Linear  diameter_pressure_gain=1.2e-6 m/MPa  wall_thickness=0.05 m  elastic_modulus=69 GPa  stress_TLU=[276, 310] MPa  strain_TLU=[.004, .02]  stress_assert_action=simscape.enum.assert.action.none  stress_max=400 MPa  poisson_ratio=0.33  wall_time_constant=0.01 s  thermal_expansion=false  alpha_L_wall=24 um/(deltaK*m)  thermal_expansion_Tref=293.15 K  heat_transfer_spec=1  mdot_nominal_heat=[ 0.1 1 ] kg/s  T_in_nominal=[ 293.15 293.15 ] K  T_out_nominal=[ 300 300 ] K  p_in_nominal_heat=[ 0.101325 0.101325 ] MPa  T_wall_nominal=[ 303.15 303.15 ] K  a_coeff=0.023  b_Re_power=0.8  c_Pr_power=0.4  Nu_lam=Cooling.MotorA1.Pipe.laminarNusselt.Value  Re_Colburn_TLU=[ 100 150 1000 ]  Colburn_factor_TLU=[ 0.019 0.013 0.002 ]  Re_Nu_TLU=[ 100 150 1000 ]  Pr_Nu_TLU=[ 1 10 ]  Nu_TLU=[ 3.72 4.21; 3.75 4.44; 4.21 7.15 ]  p0_vec=0.101325 MPa  T0_vec=300 K  mdot0=0.1 kg/s  p_nominal=0.101325 MPa  T_nominal=293.15 K
  Pump : fl_lib/Thermal Liquid/Sources/Flow Rate Source (TL)  source_type=foundation.enum.constant_controlled.controlled  flow_type=foundation.enum.mass_volumetric_flow.mass  mass_flow=0 kg/s  volumetric_flow=0 m^3/s  power_spec=foundation.enum.power_spec.isentropic  area=Cooling.Pump.area.Value m^2
  Pump Control : Subsystem
  Sensing T Amb : Subsystem
  Sensing T Conv : Subsystem
  Sensing T MotorR : Subsystem
  Simulink-PS Converter : nesl_utility/Simulink-PS Converter  PhysicalDomain=network_engine_domain  SubClassName=ps_input  LeftPortType=input  RightPortType=output  PseudoPeriodic=off  Frequencies=[]  NoiseDistribution=none  NoiseParameters=[]  Unit=kg/s  AffineConversion=off  FilteringAndDerivatives=filter  SimscapeFilterOrder=1  InputFilterTimeConstant=1  UdotUserProvided=0
  Tank : Subsystem
  Thermal Circuit Converter FC : Subsystem
  Thermal Circuit MotorA1 : Subsystem
  Thermal Liquid Properties (TL) : SimscapeFluids_lib/Thermal Liquid/Utilities/Thermal Liquid Properties (TL)  fluid_list=fluids.thermal_liquid.utilities.enum.thermal_liquid_fluid_list.ethylene_glycol  concentration_param_EG=fluids.thermal_liquid.utilities.enum.thermal_liquid_concentration.volume_fraction  concentration_param_PG=fluids.thermal_liquid.utilities.enum.thermal_liquid_concentration.volume_fraction  c_mass_SW=3.5e-3  c_mass_EG=0.1  c_mass_PG=0.1  c_mass_GL=0.1  c_vol_EG=Cooling.Fluid.rEthyleneGlycol.Value  c_vol_PG=0.1  beta_const_EG=Cooling.Fluid.bulkModulus.Value GPa  beta_const_PG=2.1791 GPa  beta_const_GL=2.1791 GPa  p_min_EG=Cooling.Fluid.pMin.Value MPa  p_min_PG=0.01 MPa  p_min_GL=0.01 MPa  p_max_EG=Cooling.Fluid.pMax.Value MPa  p_max_PG=50 MPa  p_max_GL=50 MPa  T_atm=293.15 K  p_atm=0.101325 MPa  properties_range_check=simscape.enum.assert.action.error  air_fraction=0  R_air=0.287 kJ/(K*kg)  air_dissolution_model=false  p_crit=3 MPa
  HMot : PMIOPort  Side=Left
  HConv : PMIOPort  Port=2  Side=Left
  HAmb : PMIOPort  Port=3  Side=Left
  Out Bus Element : Outport  PortName=m  Element=TCoolant
  Out Bus Element1 : Outport  PortName=m  Element=TMotorA1
  Out Bus Element2 : Outport  PortName=m  Element=TConverter
  wires:
  Sensing T Conv/1(T) -> Out Bus Element2/1
  Sensing T Amb/1(T) -> Pump Control/1(TAmb)
  Sensing T MotorR/1(T) -> Out Bus Element1/1, Pump Control/2(TMotor)
  PS-Simulink Converter/1 -> Out Bus Element/1
  Pump Control/1(Pump_flw) -> Simulink-PS Converter/1
  connections:
  HConv/RConn1 -- Sensing T Conv/LConn1 -- Thermal Circuit Converter FC/LConn1
  Tank/RConn2 -- PS-Simulink Converter/LConn1
  Sensing T MotorR/LConn1 -- Thermal Circuit MotorA1/LConn1 -- HMot/RConn1
  Thermal Circuit Converter FC/RConn1 -- Pipe Converter/LConn2
  Pump/LConn1 -- Thermal Liquid Properties (TL)/RConn1 -- Tank/RConn1
  Tank/LConn1 -- Heat Exchanger/RConn1
  Pipe Motor A1/RConn1 -- Flow Restriction MotorR HX/LConn1
  Flow Restriction Pump Converter/RConn1 -- Pipe Converter/LConn1
  Heat Exchanger/LConn1 -- Flow Restriction MotorR HX/RConn1
  Heat Exchanger/LConn2 -- Tank/LConn2 -- Tank/LConn3 -- Sensing T Amb/LConn1 -- HAmb/RConn1
  Thermal Circuit MotorA1/RConn1 -- Pipe Motor A1/LConn2
  Simulink-PS Converter/RConn1 -- Pump/LConn2
  Pump/RConn1 -- Flow Restriction Pump Converter/LConn1
  Flow Restriction Converter MotorR/LConn1 -- Pipe Converter/RConn1
  Pipe Motor A1/LConn1 -- Flow Restriction Converter MotorR/RConn1

== system ssc_car_fuel_cell_1motor/Vehicle/Powertrain/FuelCell1Motor/Battery/PowerLoss ==
  PLoss : Inport
  VBatt : Inport  Port=2
  Controlled Current Source : fl_lib/Electrical/Electrical Sources/Controlled Current Source
  Divide : Product  Inputs=*/
  Saturation : Saturate  UpperLimit=inf  LowerLimit=200
  Simulink-PS Converter : nesl_utility/Simulink-PS Converter  PhysicalDomain=network_engine_domain  SubClassName=ps_input  LeftPortType=input  RightPortType=output  PseudoPeriodic=off  Frequencies=[]  NoiseDistribution=none  NoiseParameters=[]  Unit=A  AffineConversion=off  FilteringAndDerivatives=filter  SimscapeFilterOrder=1  InputFilterTimeConstant=0.01  UdotUserProvided=0
  + : PMIOPort  Side=Left
  - : PMIOPort  Port=2  Side=Right
  wires:
  Saturation/1 -> Divide/2
  Divide/1 -> Simulink-PS Converter/1
  PLoss/1 -> Divide/1
  VBatt/1 -> Saturation/1
  connections:
  Simulink-PS Converter/RConn1 -- Controlled Current Source/RConn1
  +/RConn1 -- Controlled Current Source/RConn2
  -/RConn1 -- Controlled Current Source/LConn1

== system ssc_car_fuel_cell_1motor/Vehicle/Powertrain/FuelCell1Motor/Battery/Sensor VI ==
  Bus Creator : BusCreator  Inputs=2
  Current Sensor : fl_lib/Electrical/Electrical Sensors/Current Sensor
  PS-Simulink Converter2 : nesl_utility/PS-Simulink Converter  PhysicalDomain=network_engine_domain  SubClassName=ps_output  LeftPortType=input  RightPortType=output  PseudoPeriodic=off  Frequencies=[]  VectorFormat=1-D array  Unit=1  AffineConversion=off
  PS-Simulink Converter4 : nesl_utility/PS-Simulink Converter  PhysicalDomain=network_engine_domain  SubClassName=ps_output  LeftPortType=input  RightPortType=output  PseudoPeriodic=off  Frequencies=[]  VectorFormat=1-D array  Unit=1  AffineConversion=off
  Transfer Fcn1 : TransferFcn  Denominator=[.001 1]
  Transfer Fcn5 : TransferFcn  Denominator=[.001 1]
  Voltage Sensor2 : fl_lib/Electrical/Electrical Sensors/Voltage Sensor
  + : PMIOPort  Side=Left
  - : PMIOPort  Port=2  Side=Right
  G : PMIOPort  Port=3  Side=Right
  vi : Outport
  wires:
  Bus Creator/1 -> vi/1
  Transfer Fcn5/1 -> Bus Creator/1  "v"
  Transfer Fcn1/1 -> Bus Creator/2  "i"
  PS-Simulink Converter2/1 -> Transfer Fcn1/1
  PS-Simulink Converter4/1 -> Transfer Fcn5/1
  connections:
  Current Sensor/RConn1 -- PS-Simulink Converter2/LConn1
  Voltage Sensor2/RConn2 -- G/RConn1
  Current Sensor/RConn2 -- -/RConn1
  PS-Simulink Converter4/LConn1 -- Voltage Sensor2/RConn1
  Voltage Sensor2/LConn1 -- Current Sensor/LConn1 -- +/RConn1

== system ssc_car_fuel_cell_1motor/Vehicle/Powertrain/FuelCell1Motor/Battery/Thermal ==
  Controlled Heat Flow Rate Source : fl_lib/Thermal/Thermal Sources/Controlled Heat Flow Rate Source
  PS Gain : fl_lib/Physical Signals/Functions/PS Gain  Commented=on  gain=0.001 Ohm
  PS Math Function : fl_lib/Physical Signals/Functions/PS Math Function  Commented=on  fcn_choice=foundation.enum.math_function.square  v=1
  PS Power Function : customMath_lib/PS Power Function  resistance=Battery.Converter.resistance.Value Ohm
  Thermal Mass : fl_lib/Thermal/Thermal Elements/Thermal Mass  mass_type=foundation.enum.constant_variable.constant  mass=Battery.Converter.mThermal.Value kg  sp_heat="Battery.Converter.Cp.Value  J/kg/K"  mass_min=1e-6 kg  num_ports=foundation.enum.numPorts2.one  m_specify=off  m_priority=High  m=1 kg  m_nominal_specify=off  m_nominal_value=1  m_nominal_unit=kg  T_specify=off  T_priority=High  T=300 K  T_nominal_specify=off  T_nominal_value=1  T_nominal_unit=K  Q_specify=off  Q_priority=None  Q=0 W  Q_nominal_specify=off  Q_nominal_value=1  Q_nominal_unit=W
  Thermal Resistance : fl_lib/Thermal/Thermal Elements/Thermal Resistance  resistance=Battery.Converter.rThermal.Value K/W  T_specify=off  T_priority=None  T=0 K  T_nominal_specify=off  T_nominal_value=1  T_nominal_unit=K  Q_specify=off  Q_priority=None  Q=0 W  Q_nominal_specify=off  Q_nominal_value=1  Q_nominal_unit=W
  Thermal Reference3 : fl_lib/Thermal/Thermal Elements/Thermal Reference
  H : PMIOPort  Side=Right
  i : PMIOPort  Port=2  Side=Left
  connections:
  PS Power Function/RConn1 -- Controlled Heat Flow Rate Source/RConn1
  PS Power Function/LConn1 -- i/RConn1
  H/RConn1 -- Thermal Resistance/RConn1
  Thermal Reference3/LConn1 -- Controlled Heat Flow Rate Source/RConn2
  PS Gain/LConn1 -- PS Math Function/RConn1
  Controlled Heat Flow Rate Source/LConn1 -- Thermal Mass/LConn1 -- Thermal Resistance/LConn1

== system ssc_car_fuel_cell_1motor/Vehicle/Powertrain/FuelCell1Motor/Fuel Cell/Boost Converter Control ==
  FCcurrCMD : Inport
  FCcurr : Inport  Port=2
  Add : Sum
  Add1 : Sum  Inputs=-+
  Compare To Constant : simulink/Logic and Bit Operations/Compare To Constant  relop=<=  const=0.01  OutDataTypeStr=boolean
  Constant : Constant  Value=0
  Constant3 : Constant  Value=FuelCell.ConverterB.Control.Bias.Value
  PID Controller : slpidlib/PID Controller  Controller=PID  Form=Parallel  TimeDomain=Continuous-time  UseExternalTs=off  SampleTime=-1  IntegratorMethod=Forward Euler  FilterMethod=Forward Euler  ControllerParametersSource=internal  P=FuelCell.ConverterB.Control.P.Value  I=FuelCell.ConverterB.Control.I.Value  UseKiTs=off  D=FuelCell.ConverterB.Control.D.Value  UseExternalDerivativeSource=off  N=FuelCell.ConverterB.Control.N.Value  UseFilter=on  TunerSelectOption=Transfer Function Based (PID Tuner App)  InitialConditionSource=external  InitialConditionForIntegrator=0  InitialConditionForFilter=0  DifferentiatorICPrevScaledInput=0  ExternalReset=falling  TrackingMode=off  Kt=1  LimitOutput=on  SatLimitsSource=internal  UpperSaturationLimit=1  LowerSaturationLimit=-1  LinearizeAsGain=on  AntiWindupMode=clamping  Kb=1  LimitIntegrator=off  UpperIntegratorSaturationLimit=inf  LowerIntegratorSaturationLimit=-inf  POutMin=[]  POutMax=[]  IOutMin=[]  IOutMax=[]  DOutMin=[]  DOutMax=[]  NOutMin=[]  NOutMax=[]  SumOutMin=[]  SumOutMax=[]  SaturationOutMin=[]  SaturationOutMax=[]  PParamMin=[]  PParamMax=[]  IParamMin=[]  IParamMax=[]  DParamMin=[]  DParamMax=[]  NParamMin=[]  NParamMax=[]  KbParamMin=[]  KbParamMax=[]  KtParamMin=[]  KtParamMax=[]  KbOutMin=[]  KbOutMax=[]  KtOutMin=[]  KtOutMax=[]  IntegratorOutMin=[]  IntegratorOutMax=[]  FilterOutMin=[]  FilterOutMax=[]  SumI1OutMin=[]  SumI1OutMax=[]  SumI2OutMin=[]  SumI2OutMax=[]  SumI3OutMin=[]  SumI3OutMax=[]  SumI4OutMin=[]  SumI4OutMax=[]  SumDOutMin=[]  SumDOutMax=[]  DifferentiatorOutMin=[]  DifferentiatorOutMax=[]  FilterDiffOutCoefMin=[]  FilterDiffOutCoefMax=[]  ReciprocalOutMin=[]  ReciprocalOutMax=[]  SumDenOutMin=[]  SumDenOutMax=[]  SumNumOutMin=[]  SumNumOutMax=[]  DivideOutMin=[]  DivideOutMax=[]  UdiffTsProdOutMin=[]  UdiffTsProdOutMax=[]  NTsProdOutMin=[]  NTsProdOutMax=[]  UintegralTsProdOutMin=[]  UintegralTsProdOutMax=[]  UngainTsProdOutMin=[]  UngainTsProdOutMax=[]  ClampingZeroOutDataTypeStr=Inherit: Inherit via back propagation  ClampingZeroOutMin=[]  ClampingZeroOutMax=[]  FilterDenConstantOutDataTypeStr=Inherit: Inherit via back propagation  FilterDenConstantOutMin=[]  FilterDenConstantOutMax=[]  PCopyOutDataTypeStr=Inherit: Inherit via back propagation  PCopyOutMin=[]  PCopyOutMax=[]  NCopyOutDataTypeStr=Inherit: Inherit via back propagation  NCopyOutMin=[]  NCopyOutMax=[]  IntegratorContinuousStateAttributes=''  IntegratorStateMustResolveToSignalObject=off  IntegratorRTWStateStorageClass=Auto  FilterContinuousStateAttributes=''  FilterStateMustResolveToSignalObject=off  FilterRTWStateStorageClass=Auto  ParallelPVariant=InternalParameters  IdealPVariant=Disabled  IVariant=InternalParameters  DVariant=InternalParameters  IntegratorVariant=Continuous  SatVariant=Enabled  AWVariant=ContClampingParallel  PCopyVariant=Disabled  TRVariant=Disabled  FdbkBlocksVariant=Forward  IdealPFdbkVariant=Disabled  SatFdbkVariant=Disabled  DerivativeFilterVariant=ContFilter  NVariant=InternalParameters  NCopyVariant=Disabled  FilterICVariant=ExternalICs  IntegratorICVariant=ExternalICs  ExternalResetVariant=ExternalReset  TRSumVariant=Passthrough  SumFdbkVariant=Disabled  SumVariant=Sum_PID  TsampFilterVariant=InternalTs  TsampNgainVariant=Passthrough  TsampIntegralVariant=Disabled_SignalSpec  ExternalSaturationOutDataTypeStr=Inherit: Same as second input  DerivativeSourceVariant=ErrorSignal  PreIntVariant=InternalPreInt
  Saturation : Saturate  UpperLimit=1  LowerLimit=0  ZeroCross=off
  Transfer Fcn (with initial outputs) : simulink_extras/Additional Linear/Transfer Fcn (with initial outputs)  N=[1]  D=[FuelCell.ConverterB.Control.TFiltI0.Value 1]  Y0=0.05  U0=0
  u_boost : Outport
  wires:
  Compare To Constant/1 -> PID Controller/2
  Constant/1 -> PID Controller/4
  Transfer Fcn (with initial outputs)/1 -> PID Controller/3
  Add1/1 -> PID Controller/1
  FCcurrCMD/1 -> Add1/2, Compare To Constant/1
  Add/1 -> Saturation/1
  FCcurr/1 -> Add1/1
  PID Controller/1 -> Add/1, Transfer Fcn (with initial outputs)/1
  Saturation/1 -> u_boost/1
  Constant3/1 -> Add/2
